simulink model "MyRMS_test"  (R2024a)
settings: Solver=VariableStepAuto  StartTime=0.0  StopTime=1  RelTol=1e-3
undefined symbols (not defined in the file or in its folder): SAMPLING_FREQ
settings Model: Creator=Jan Rosa  LastModifiedBy=Jan Rosa

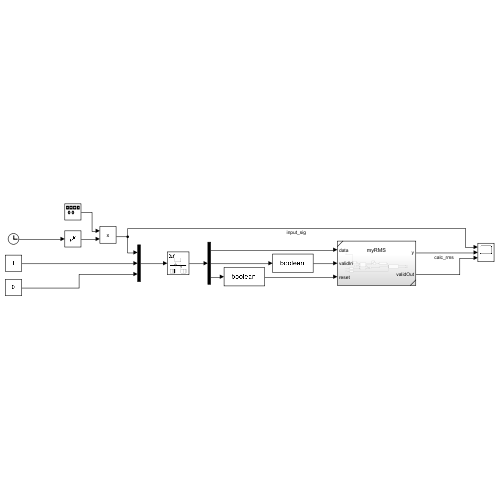
[thumbnail: Simulink's stored preview of the top-level diagram]
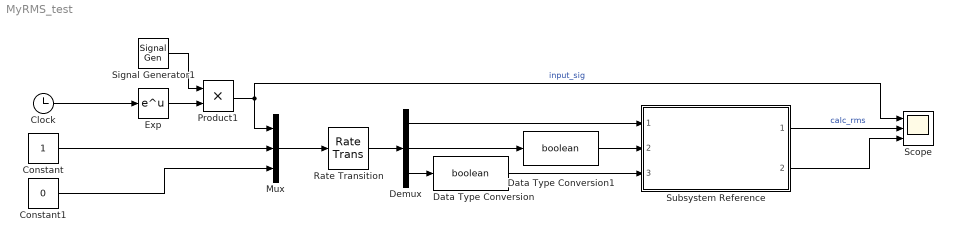
== system MyRMS_test ==
  Clock : Clock
  Constant : Constant
  Constant1 : Constant  Value=0
  Data Type Conversion : DataTypeConversion  OutDataTypeStr=boolean  SaturateOnIntegerOverflow=off  RndMeth=Floor
  Data Type Conversion1 : DataTypeConversion  OutDataTypeStr=boolean  SaturateOnIntegerOverflow=off  RndMeth=Floor
  Demux : Demux  Outputs=3
  Exp : Math
  Mux : Mux  Inputs=3
  Product1 : Product
  Rate Transition : RateTransition  Deterministic=off  OutPortSampleTime=1/SAMPLING_FREQ
  Scope : Scope  NumInputPorts=3
  Signal Generator1 : SignalGenerator  Frequency=50
  Subsystem Reference : Subsystem  ReferencedSubsystem=myRMS
  wires:
  Constant1/1 -> Mux/3
  Constant/1 -> Mux/2
  Product1/1 -> Scope/1, Mux/1  "input_sig"
  Subsystem Reference/1 -> Scope/2  "calc_rms"
  Subsystem Reference/2 -> Scope/3
  Mux/1 -> Rate Transition/1
  Demux/1 -> Subsystem Reference/1
  Demux/2 -> Data Type Conversion1/1
  Demux/3 -> Data Type Conversion/1
  Rate Transition/1 -> Demux/1
  Data Type Conversion/1 -> Subsystem Reference/3
  Data Type Conversion1/1 -> Subsystem Reference/2
  Clock/1 -> Exp/1
  Exp/1 -> Product1/2
  Signal Generator1/1 -> Product1/1
